simulink model "battery_pack_cooling"  (R2021a)
settings: Solver=FixedStepAuto  StartTime=0.0  StopTime=1400  FixedStep=1  RelTol=1e-3
values from neighbouring files (symbols this model uses):
  Bc = 810.5328    [imports_battery_cooling.m]
  c = 1350    [imports_battery_cooling.m]
  Cell_length = 0.227    [imports_battery_cooling.m]
  Cell_Voltage = Cell(:,2:3)    [imports_battery_cooling.m]
  Cell_width = 0.226    [imports_battery_cooling.m]
  Cr = [0.0117,0.0085,0.0090 ... (first row only)    [imports_battery_cooling.m]
  h_conv = 5    [imports_battery_cooling.m]
  Mb = 150.2    [imports_battery_cooling.m]
  Np = 2    [imports_battery_cooling.m]
  Ns = 96    [imports_battery_cooling.m]
  Ri = 0.0023    [imports_battery_cooling.m]
  SOC = [0;0.1;0.25;0.5;0.75;0.9;1.0]    [imports_battery_cooling.m]
  T = [278.15;293.15;313.15]    [imports_battery_cooling.m]
  Tamb = 293.15    [imports_battery_cooling.m]    (also in imports_motor_cooling.m = 18)
settings Model: Creator=shubh  LastModifiedBy=shubh

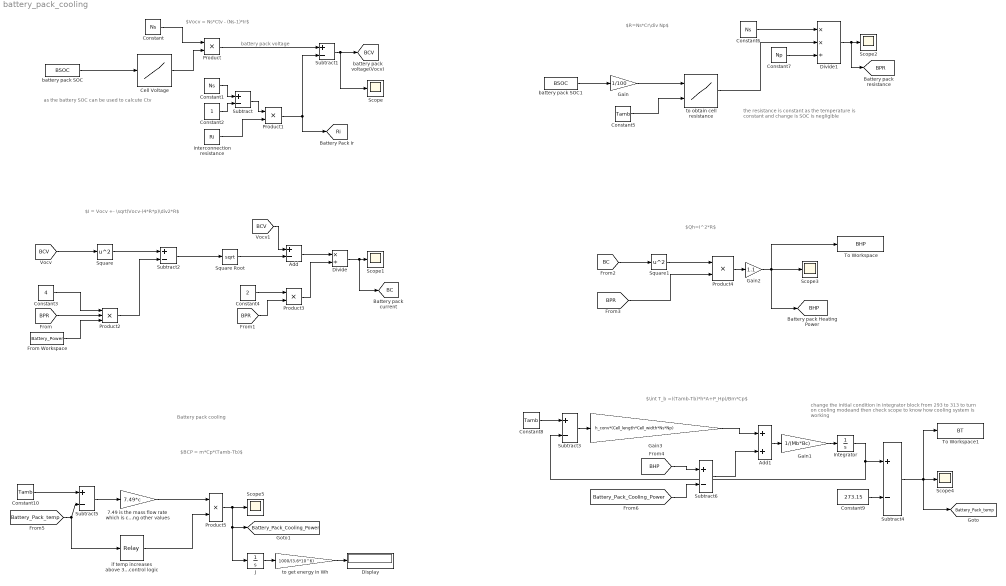
== system battery_pack_cooling ==
  note: change the initial condition in integrator block from 293 to 313
      | to turn on cooling modeand then check scope to know how cooling
      | system is working
  note: $BCP = m*Cp*(Tamb-Tb)$
  note: Battery pack cooling
  note: $\int T_b =((Tamb-Tb)*h*A+P_Hp)/Bm*Cp$
  note: the resistance is constant as the temperature is constant and change is SOC is negligible
  note: battery pack voltage
  note: as the battery SOC can be used to calcute Ctv
  note: $Vocv = Ns*Ctv - (Ns-1)*Ir$
  note: $I = Vocv +- \sqrt(Vocv-(4*R*p)\div2*R$
  note: $R=Ns*Cr\div Np$
  note: $Qh=I^2*R$
  7.49 is the mass flow rate which is calculated by taking bcp =bhp*1.1 and putting other values : Gain  Gain=7.49*c
  Add : Sum  Inputs=+-
  Add1 : Sum
  "Cell Voltage " : Lookup_n-D  NumberOfTableDimensions=1  BreakpointsForDimension1=Cell_Voltage( :,2)  Table=Cell_Voltage( :,1)  InternalRulePriority=Speed  RndMeth=Simplest  InputSameDT=on
  Constant : Constant  Value=Ns
  Constant1 : Constant  Value=Ns
  Constant10 : Constant  Value=Tamb
  Constant2 : Constant
  Constant3 : Constant  Value=4
  Constant4 : Constant  Value=2
  Constant5 : Constant  Value=Tamb
  Constant6 : Constant  Value=Ns
  Constant7 : Constant  Value=Np
  Constant8 : Constant  Value=Tamb
  Constant9 : Constant  Value=273.15
  Display : Display
  Divide : Product  Inputs=*/
  Divide1 : Product  Inputs=**/
  From Workspace : FromWorkspace  VariableName=Battery_Power
  Gain : Gain  Gain=1/100
  Gain1 : Gain  Gain=1/(Mb*Bc)
  Gain2 : Gain  Gain=1.1
  Gain3 : Gain  Gain=h_conv*(Cell_length*Cell_width*Ns*Np)
  Integrator : Integrator  InitialCondition=313.17
  J : Integrator
  Product{,1,3..5} (5 alike) : Product
  Product2 : Product  Inputs=3
  Scope{,1..5} (6 alike) : Scope
  Square : Math  Operator=square  SaturateOnIntegerOverflow=on
  Square Root : Sqrt  SaturateOnIntegerOverflow=on
  Square1 : Math  Operator=square  SaturateOnIntegerOverflow=on
  Subtract{,1..6} (7 alike) : Sum  Inputs=+-
  To Workspace : ToWorkspace  VariableName=BHP  SaveFormat=Timeseries  SampleTime=-1
  To Workspace1 : ToWorkspace  VariableName=BT  SaveFormat=Timeseries  SampleTime=-1
  battery pack SOC : FromWorkspace  VariableName=BSOC
  battery pack SOC1 : FromWorkspace  VariableName=BSOC
  if temp increases above 30 then cooling is turned on and output is 1 else 0 is send as output if temp is b/w 20 and 30 or lower than that it works as a control logic : Relay  OnSwitchValue=30  OffSwitchValue=20
  interconnection resistance : Constant  Value=Ri
  to get energy in Wh : Gain  Gain=1000/(3.6*10^6)
  "to obtain cell resistance " : Lookup_n-D  BreakpointsForDimension1=SOC  BreakpointsForDimension2=T  Table=Cr  InternalRulePriority=Speed  RndMeth=Simplest  InputSameDT=on
      settings: InputPortMap=u0,u1
  tag scope: BC=global, BCV=global, BHP=global, BPR=global, Battery_Pack_Cooling_Power=global, Battery_Pack_temp=global, Ri=global
  wires:
  battery pack SOC/1 -> "Cell Voltage "/1
  Constant/1 -> Product/1
  "Cell Voltage "/1 -> Product/2
  Constant1/1 -> Subtract/1
  Constant2/1 -> Subtract/2
  Subtract/1 -> Product1/1
  interconnection resistance/1 -> Product1/2
  Product/1 -> Subtract1/1
  Product1/1 -> [Ri], Subtract1/2
  Subtract1/1 -> Scope/1, [BCV]
  From Workspace/1 -> Product2/3
  [BPR] -> Product2/2
  Constant3/1 -> Product2/1
  [BCV] -> Square/1
  Square/1 -> Subtract2/1
  Product2/1 -> Subtract2/2
  Subtract2/1 -> Square Root/1
  Square Root/1 -> Add/2
  [BPR] -> Product3/2
  Constant4/1 -> Product3/1
  Product3/1 -> Divide/2
  Divide/1 -> [BC], Scope1/1
  [BCV] -> Add/1
  Add/1 -> Divide/1
  battery pack SOC1/1 -> Gain/1
  Gain/1 -> "to obtain cell resistance "/1
  Constant5/1 -> "to obtain cell resistance "/2
  "to obtain cell resistance "/1 -> Divide1/2
  Constant6/1 -> Divide1/1
  Constant7/1 -> Divide1/3
  Divide1/1 -> [BPR], Scope2/1
  [BC] -> Square1/1
  Square1/1 -> Product4/1
  [BPR] -> Product4/2
  Gain2/1 -> To Workspace/1, [BHP], Scope3/1
  Add1/1 -> Gain1/1
  [BHP] -> Subtract6/1
  Gain1/1 -> Integrator/1
  Integrator/1 -> Subtract4/1, Subtract3/2
  Product4/1 -> Gain2/1
  Constant8/1 -> Subtract3/1
  Subtract3/1 -> Gain3/1
  Gain3/1 -> Add1/1
  Subtract4/1 -> [Battery_Pack_temp], To Workspace1/1, Scope4/1
  Constant9/1 -> Subtract4/2
  Constant10/1 -> Subtract5/1
  [Battery_Pack_temp] -> if temp increases above 30 then cooling is turned on and output is 1 else 0 is send as output if temp is b/w 20 and 30 or lower than that it works as a control logic/1, Subtract5/2
  Subtract5/1 -> 7.49 is the mass flow rate which is calculated by taking bcp =bhp*1.1 and putting other values/1
  7.49 is the mass flow rate which is calculated by taking bcp =bhp*1.1 and putting other values/1 -> Product5/1
  if temp increases above 30 then cooling is turned on and output is 1 else 0 is send as output if temp is b/w 20 and 30 or lower than that it works as a control logic/1 -> Product5/2
  Product5/1 -> Scope5/1, J/1, [Battery_Pack_Cooling_Power]
  [Battery_Pack_Cooling_Power] -> Subtract6/2
  Subtract6/1 -> Add1/2
  J/1 -> to get energy in Wh/1
  to get energy in Wh/1 -> Display/1
